simulink model "xplane2matlab"  (R2016a)
settings: Solver=ode45  StartTime=0.0  StopTime=inf  RelTol=1e-3
libraries: xpcutilitieslib x2, xpcobsoletelib x2, instrumentlib x2, simulink x1
settings Model: Creator=IEE12  LastModifiedBy=Marcelo
settings DataIOCC: LimitDataPoints=on  SaveFormat=Array
settings DebuggingCC: UnderspecifiedInitializationDetection=Classic  MergeDetectMultiDrivingBlocksExec=none  SolverPrmCheckMsg=warning  StateNameClashWarn=warning
settings HardwareCC: ProdBitPerPointer=32  ProdLargestAtomicFloat=None  ProdIntDivRoundTo=Undefined  ProdEndianess=Unspecified  ProdWordSize=32  ProdHWDeviceType=32-bit Generic
settings ModelReferenceCC: PropagateSignalLabelsOutOfModel=off
settings ConfigComp: CovModelRefEnable=Off

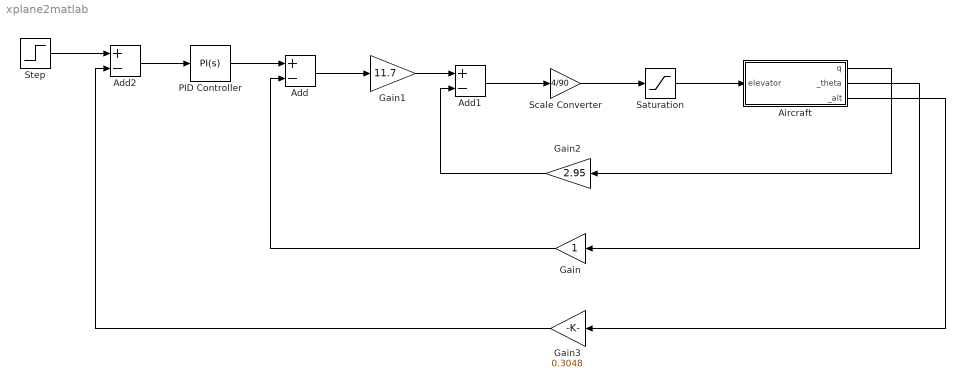
== system xplane2matlab ==
  Add : Sum  Inputs=+-
  Add1 : Sum  Inputs=+-
  Add2 : Sum  Inputs=+-
  Aircraft : Subsystem
  Gain : Gain
  Gain1 : Gain  Gain=11.7
  Gain2 : Gain  Gain=2.95
  Gain3 : Gain  Gain=0.3048
  PID Controller : simulink/Continuous/PID Controller  Controller=PI  TimeDomain=Continuous-time  SampleTime=-1  IntegratorMethod=Forward Euler  FilterMethod=Forward Euler  Form=Parallel  UseFilter=on  ControllerParametersSource=internal  P=0.000674  I=4.28e-06  D=0  N=100  InitialConditionSource=internal  InitialConditionForIntegrator=0  InitialConditionForFilter=0  ExternalReset=none  LimitOutput=off  UpperSaturationLimit=inf  LowerSaturationLimit=-inf  LinearizeAsGain=on  AntiWindupMode=none  Kb=1  TrackingMode=off  Kt=1  PParamMin=[]  PParamMax=[]  IParamMin=[]  IParamMax=[]  DParamMin=[]  DParamMax=[]  NParamMin=[]  NParamMax=[]  KbParamMin=[]  KbParamMax=[]  KtParamMin=[]  KtParamMax=[]  POutMin=[]  POutMax=[]  IOutMin=[]  IOutMax=[]  DOutMin=[]  DOutMax=[]  NOutMin=[]  NOutMax=[]  KbOutMin=[]  KbOutMax=[]  KtOutMin=[]  KtOutMax=[]  IntegratorOutMin=[]  IntegratorOutMax=[]  FilterOutMin=[]  FilterOutMax=[]  SumOutMin=[]  SumOutMax=[]  SumI1OutMin=[]  SumI1OutMax=[]  SumI2OutMin=[]  SumI2OutMax=[]  SumI3OutMin=[]  SumI3OutMax=[]  SumDOutMin=[]  SumDOutMax=[]  SaturationOutMin=[]  SaturationOutMax=[]  IntegratorContinuousStateAttributes=''  IntegratorStateMustResolveToSignalObject=off  IntegratorRTWStateStorageClass=Auto  FilterContinuousStateAttributes=''  FilterStateMustResolveToSignalObject=off  FilterRTWStateStorageClass=Auto  DifferentiatorICPrevScaledInput=0  DifferentiatorOutMin=[]  DifferentiatorOutMax=[]
  Saturation : Saturate  UpperLimit=1.0  LowerLimit=-1.0
  Scale Converter : Gain  Gain=4/90
  Step : Step  After=8000*0.3048  SampleTime=0
  wires:
  Gain/1 -> Add/2
  Add/1 -> Gain1/1
  Gain1/1 -> Add1/1
  Gain2/1 -> Add1/2
  Aircraft/2("_theta ") -> Gain/1
  Add1/1 -> Scale Converter/1
  Aircraft/1("q ") -> Gain2/1
  Saturation/1 -> Aircraft/1(elevator)
  Scale Converter/1 -> Saturation/1
  PID Controller/1 -> Add/1
  Step/1 -> Add2/1
  Aircraft/3(_alt) -> Gain3/1
  Add2/1 -> PID Controller/1
  Gain3/1 -> Add2/2

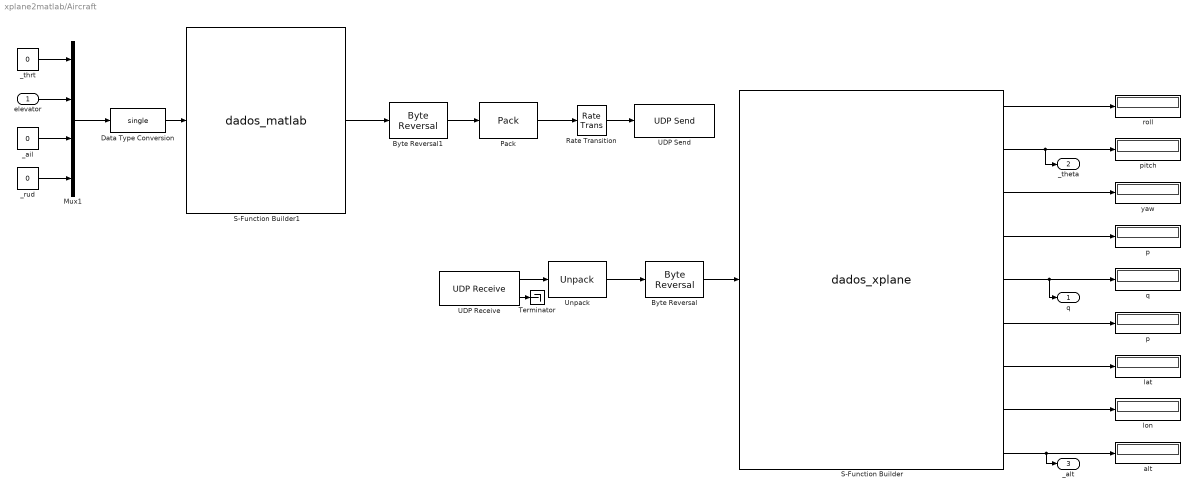
== system xplane2matlab/Aircraft ==
  elevator : Inport
  Byte Reversal : xpcutilitieslib/Byte Reversal   numInp=1
  Byte Reversal1 : xpcutilitieslib/Byte Reversal   numInp=1
  Data Type Conversion : DataTypeConversion  OutDataTypeStr=single
  Mux1 : Mux
  Pack : xpcobsoletelib/Utilities/Pack   datatypes={'uint8'}  byteAlign=1
  Rate Transition : RateTransition  OutPortSampleTime=0.05
  S-Function Builder : S-Function  InitFcn=try, set_param(gcb,'FunctionName','dados_xplane'), end  FunctionName=dados_xplane  SFunctionModules=dados_xplane_wrapper  SFunctionDeploymentMode=off  EnableBusSupport=off  mask(S-Function Builder){}
      mask help: Simulink:masks:SFunctionBuilder_MD
      mask init:
      | val = [[.9  0.75 0.75 1 1 .9 .9 1]',[1 1 0.75 0.75 .9 .9 1 .9]'];try , sys = get_param(gcb,'SfunBuilderFcnName');if isempty(sys), sys = get_param(gcb,'FunctionName'); end,catch, sys = get_param(gcb,'FunctionName'); end
      settings: CopyFcn=set_param(gcbh,'LinkStatus','none')  PreSaveFcn=try, set_param(gcb,'FunctionName','dados_xplane'), end  OpenFcn=sfunctionwizard(gcbh)
      mask Display: plot(val(:,1),val(:,2)),disp(sys), port_label('input',1,'Pkt'), port_label('output',1,'phi'), port_label('output',2,'theta'), port_label('output',3,'psi'), port_label('output',4,'p'), port_label('output',5,'q'), port_label('output',6,'r'), port_label('output',7,'lat'), port_label('output',8,'lon'), port_label('output',9,'alt')
  S-Function Builder1 : S-Function  InitFcn=try, set_param(gcb,'FunctionName','dados_matlab'), end  FunctionName=dados_matlab  SFunctionModules=dados_matlab_wrapper  SFunctionDeploymentMode=off  EnableBusSupport=off  mask(S-Function Builder){}
      mask help: Simulink:masks:SFunctionBuilder_MD
      mask init: same as xplane2matlab/Aircraft/S-Function Builder
      settings: CopyFcn=set_param(gcbh,'LinkStatus','none')  PreSaveFcn=try, set_param(gcb,'FunctionName','dados_matlab'), end  OpenFcn=sfunctionwizard(gcbh)
      mask Display: plot(val(:,1),val(:,2)),disp(sys), port_label('input',1,'du'), port_label('output',1,'Pkt')
  Terminator : Terminator
  UDP Receive : instrumentlib/UDP Receive  Host=127.0.0.1  Port=49001  LocalPort=49004  DataSize=149  EnableBlockingMode=off  Timeout=10  SampleTime=0.05  DataType=uint8  ByteOrder=BigEndian
  UDP Send : instrumentlib/UDP Send  Host=127.0.0.1  Port=49000  LocalPort=-1  EnableBlockingMode=on  ByteOrder=BigEndian
  Unpack : xpcobsoletelib/Utilities/Unpack   dimensions={[1 149]}  datatypes={'uint8'}  byteAlign=1
  _ail : Constant  Value=0
  _rud : Constant  Value=0
  _thrt : Constant  Value=0
  alt : Display
      settings: Format=bank
  "lat " : Display
      settings: Format=bank
  lon : Display
      settings: Format=bank
  p : Display
      settings: Format=bank
  "p " : Display
      settings: Format=bank
  pitch : Display
      settings: Format=bank
  q : Display
      settings: Format=bank
  roll : Display
      settings: Format=bank
  "yaw " : Display
      settings: Format=bank
  "q " : Outport
  "_theta " : Outport  Port=2
  _alt : Outport  Port=3
  wires:
  UDP Receive/2 -> Terminator/1
  UDP Receive/1 -> Unpack/1
  Unpack/1 -> Byte Reversal/1
  Byte Reversal/1 -> S-Function Builder/1
  S-Function Builder/3 -> "yaw "/1
  S-Function Builder/4 -> "p "/1
  S-Function Builder/5 -> "q "/1, q/1
  S-Function Builder/9 -> _alt/1, alt/1
  Byte Reversal1/1 -> Pack/1
  S-Function Builder1/1 -> Byte Reversal1/1
  Data Type Conversion/1 -> S-Function Builder1/1
  Pack/1 -> Rate Transition/1
  Rate Transition/1 -> UDP Send/1
  Mux1/1 -> Data Type Conversion/1
  _rud/1 -> Mux1/4
  _thrt/1 -> Mux1/1
  _ail/1 -> Mux1/3
  elevator/1 -> Mux1/2
  S-Function Builder/6 -> p/1
  S-Function Builder/7 -> "lat "/1
  S-Function Builder/8 -> lon/1
  S-Function Builder/1 -> roll/1
  S-Function Builder/2 -> "_theta "/1, pitch/1
